simulink model "barra1Bode"  (R2018a)
settings: Solver=ode45  StartTime=0.0  StopTime=100  RelTol=1e-6  EnableMultiTasking=on
InitFcn:
  | barrassmodel=load('/Users/leonardopedroso/Desktop/CComp/Lab/1_identification/model/barrassmodel.mat');
StopFcn:
  | [trueMag,truePhase,w]=bode(sys.values);semilogx(squeeze(w),20*log10(squeeze(trueMag)))
  | subplot(211)
  | semilogx(squeeze(w),20*log10(squeeze(trueMag)))
  | subplot(212)
  | semilogx(squeeze(w),squeeze(truePhase))
  | save('./DATA/bodeData.mat','trueMag','truePhase','w');
  | clear;
libraries: slctrlblks x1
settings Model: Creator=jomle  LastModifiedBy=leonardopedroso
settings DataIOCC: LimitDataPoints=on  SaveFormat=Array
settings OptimizationCC: LifeSpan=inf
settings DebuggingCC: SFUnexpectedBacktrackingDiag=warning  SFNoUnconditionalDefaultTransitionDiag=warning  SFExecutionAtInitializationDiag=none
settings HardwareCC: ProdBitPerPointer=32  ProdBitPerSizeT=32  ProdBitPerPtrDiffT=32  ProdLargestAtomicFloat=None  ProdIntDivRoundTo=Undefined  ProdEndianess=Unspecified  ProdWordSize=32  ProdHWDeviceType=32-bit Generic
settings ModelReferenceCC: PropagateSignalLabelsOutOfModel=off
settings CodeAppCC: StateflowObjectComments=on
settings GRTTargetCC: TargetLangStandard=C89/C90 (ANSI)  GeneratePreprocessorConditionals=Disable all
settings ConfigComp: CovMetricSettings=dw  CovHtmlReporting=on  CovSaveCumulativeToWorkspaceVar=on  CovSaveSingleToWorkspaceVar=on  CovExternalEMLEnable=off

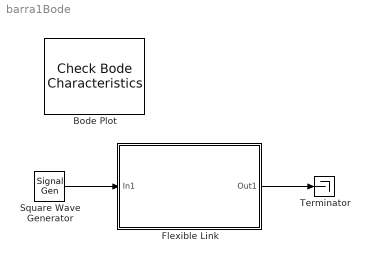
== system barra1Bode ==
  Bode Plot : slctrlblks/Model Verification/Check Bode  Characteristics  InstantiateOnLoad=on  SaveOperatingPoints=off  LinearizationIOs={'/Flexible Link', 1, 'out', 'off', '';'/Square Wave Generator', 1, 'in', 'on', ''}  LinearizeAt=SnapshotTimes  SnapshotTimes=[0]  TriggerType=rising  SampleTime=auto  RateConversionMethod=zoh  PreWarpFreq=10  UseExactDelayModel=off  UseFullBlockNameLabels=off  UseBusSignalLabels=off  enabled=on  stopWhenAssertionFail=off  export=off  ViewDlgPos=[510 1259 510 390]  OpenViewOnLoad=off  LaunchViewOnOpen=off  FrequencyUnits=rad/s  MagnitudeUnits=dB  PhaseUnits=deg  TimeUnits=seconds  EnableUpperBound=off  UpperBoundFrequencies=[]  UpperBoundMagnitudes=[]  EnableLowerBound=off  LowerBoundFrequencies=[]  LowerBoundMagnitudes=[]
      settings: SourceProductName=Simulink Control Design  SaveToWorkspace=on
  Flexible Link : Subsystem
      mask Display: image('./model/quanserlink.jpg');
  Square Wave Generator : SignalGenerator  WaveForm=square  Frequency=0.2  Units=rad/sec
  Terminator : Terminator
  wires:
  Square Wave Generator/1 -> Flexible Link/1(In1)
  Flexible Link/1(Out1) -> Terminator/1

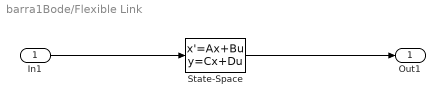
== system barra1Bode/Flexible Link ==
  In1 : Inport
  State-Space : StateSpace  A=barrassmodel.Atrue  B=barrassmodel.Btrue  C=barrassmodel.Ctrue  D=barrassmodel.Dtrue  InitialCondition=0
  Out1 : Outport
  wires:
  State-Space/1 -> Out1/1
  In1/1 -> State-Space/1
